simulink model "model_sim"  (Simulink 7.7)
settings: Solver=ode1  StartTime=0.0  StopTime=30  FixedStep=0.01  RelTol=1e-3
values from neighbouring files (symbols this model uses):
  sys = ss(A,B,C,D)    [model0001.m]
undefined symbols (not defined in the file or in its folder): Ainit, Binit, d1, DiscIntNeverNeededParam, sigbuilder_block, Tc
libraries: simulink x5
settings Model: Creator=User  LastModifiedBy=User
settings DataIOCC: LimitDataPoints=off  SaveFormat=StructureWithTime  SaveOutput=off  SignalLogging=off  DSMLogging=off  SaveTime=off

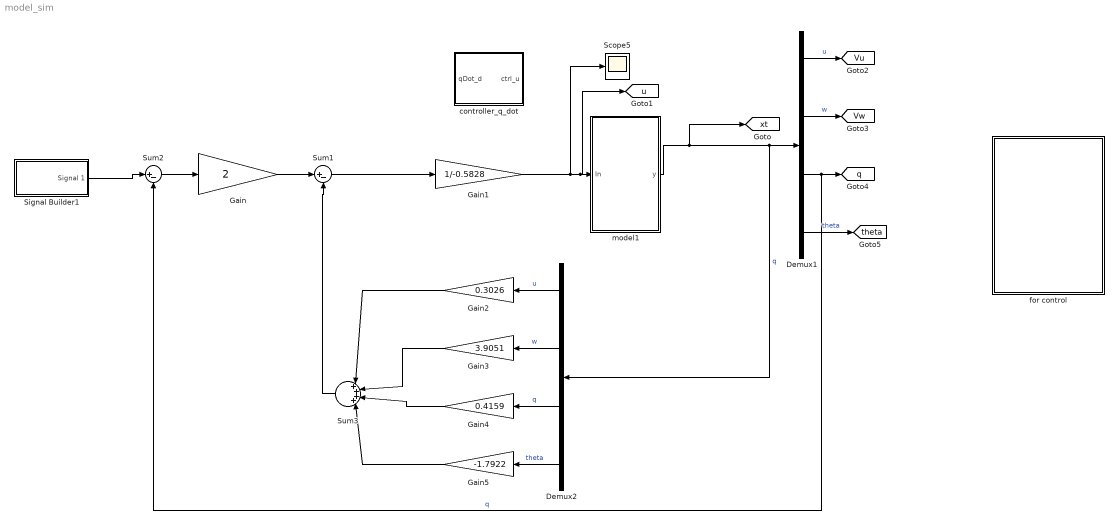
== system model_sim ==
  Demux1 : Demux
  Demux2 : Demux
  Gain : Gain  Gain=2
  Gain1 : Gain  Gain=1/-0.5828
  Gain2 : Gain  Gain=0.3026
  Gain3 : Gain  Gain=3.9051
  Gain4 : Gain  Gain=0.4159
  Gain5 : Gain  Gain=-1.7922
  Scope5 : Scope
      settings: YMin=-0.44624  YMax=0.2748
  Signal Builder1 : Subsystem  Tag=STV Subsys  LoadFcn=sigbuilder_block('load');  StartFcn=sigbuilder_block('start');  StopFcn=sigbuilder_block('stop');  ClipboardFcn=sigbuilder_block('clipboard');  mask(Sigbuilder block){}
      mask help: Create and generate interchangeable groups of signals whose waveforms are piecewise linear.
      mask init:
      | if ~strcmp(get_param(bdroot(gcbh),'SimulationStatus'),'stopped') tuvar = sigbuilder_block('maskInit'); end
      settings: CopyFcn=sigbuilder_block('copy');  DeleteFcn=sigbuilder_block('delete');  ModelCloseFcn=sigbuilder_block('modelClose');  PreSaveFcn=sigbuilder_block('preSave');  NameChangeFcn=sigbuilder_block('namechange');  OpenFcn=sigbuilder_block('open',[136.552 87.5172 549.931 396 ]);  CloseFcn=sigbuilder_block('close');
      mask Display: plot(0, 0, 100, 100,[2, 2, 32, 32, 2], [68, 8, 8, 68, 68],[32, 2], [38, 38], [32, 19, 2],[53, 60, 44], [32, 17, 17, 2],[16, 16, 31, 31]);txt = getActiveGroup(gcbh);text(2, 100, txt,'verticalAlignment', 'top');
  Sum1 : Sum  Inputs=|+-
  Sum2 : Sum  Inputs=|+-
  Sum3 : Sum  Inputs=|++++|
  controller_q_dot : Subsystem
  for control : Subsystem
  model1 : Subsystem
  tag scope: Vu=global, Vw=global, q=global, theta=global, u=global, xt=global
  wires:
  Demux1/2 -> [Vw]  "w"
  Demux2/3 -> Gain4/1  "q"
  Gain2/1 -> Sum3/1
  Demux2/1 -> Gain2/1  "u"
  Gain4/1 -> Sum3/3
  Gain5/1 -> Sum3/4
  Gain3/1 -> Sum3/2
  Demux2/4 -> Gain5/1  "theta"
  Demux1/1 -> [Vu]  "u"
  Sum2/1 -> Gain/1
  model1/1(y) -> [xt], Demux1/1, Demux2/1  "q"
  Demux2/2 -> Gain3/1  "w"
  Demux1/3 -> Sum2/2, [q]  "q"
  Demux1/4 -> [theta]  "theta"
  Gain/1 -> Sum1/1
  Sum3/1 -> Sum1/2
  Sum1/1 -> Gain1/1
  Signal Builder1/1(Signal 1) -> Sum2/1
  Gain1/1 -> [u], model1/1(In), Scope5/1

== system model_sim/Signal Builder1 ==
  Demux : Demux  Tag=STV Demux  Outputs=1
  FromWs : FromWorkspace  Tag=STV FromWs  VariableName=tuvar  SampleTime=0  SigBuilderData=DataTag0  VnvData=DataTag1
      SigBuilderData=|
      | common.afterFinalStr = 'Extrapolate'
      | common.sampleTime = 0
      | dataSet.timeRange = [0 30]
      | dataSet.name = 'Group 1'
      | sbobj.Groups.Name = 'Group 1'
      | sbobj.Groups.Signals.Name = 'Signal 1'
      | sbobj.Groups.Signals.XData = [0 0.6 0.6 1.25 1.25 1.8 1.8 2.65 2.65 3.25 3.25 3.75 3.75 4.3 4.3 5.1 5.1 6 6 6.55 6.55 7.85 7.85 8.3 8.3 8.95 8.95 9.45 9.45 10.3 10.3 10.95 10.95 11.6 11.6 12.05 12.05 13.15 13.15 14.1 14.1 15.15 15.15 15.85 15.85 16.25 16.75 17.6 18.1 18.1 19.15 19.15 19.8 19.8 20.45 20.45 21.3 21.3 21.95 21.95 23.05 23.05 23.85 23.85 24.5 24.5 25.15 25.15 25.6 25.6 26.2 26.2 26.65 26.65 27.2 27.2 27.95 27.95 28.6 28.6 29.25 29.25 30]
      | sbobj.Groups.Signals.YData = [-0.4 -0.4 -0.105 -0.105 0.53 0.53 0.17 0.17 -0.075 -0.075 0.26 0.26 -0.33 -0.33 0.055 0.055 0.405 0.405 0.29 0.29 0.255 0.255 -0.05 -0.05 0.39 0.39 -0.25 -0.25 0.135 0.135 -0.345 -0.345 -0.055 -0.055 0.19 0.19 0.31 0.31 0.445 0.445 0 0 -0.28 -0.28 0.12 0.115 0.245 -0.02 0 -0.53 -0.53 0.46 0.46 -0.11 -0.11 0.01 0.01 0.1 0.1 0.5 0.5 -0.19 -0.19 0.24 0.24 -0.09 -0.09 0 0 -0.355 -0.355 -0.115 -0.115 0.065 0.065 0.025 0.025 -0.16 -0.16 0.075 0.075 -0.04 -0.04]
      | sbobj.Groups.TimeRange = [0 30]
  Signal 1 : Outport  Tag=STV Outport
  wires:
  FromWs/1 -> Demux/1
  Demux/1 -> Signal 1/1

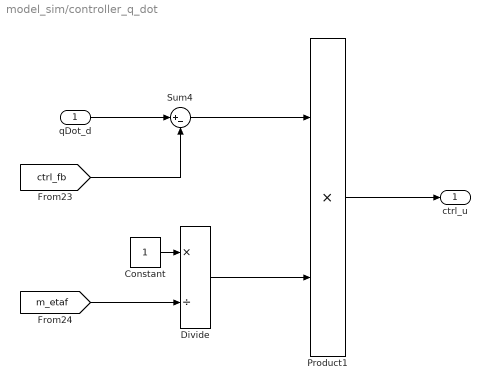
== system model_sim/controller_q_dot ==
  qDot_d : Inport
  Constant : Constant
  Divide : Product  Inputs=*/
  Product1 : Product
  Sum4 : Sum  Inputs=|+-
  ctrl_u : Outport
  wires:
  Sum4/1 -> Product1/1
  Product1/1 -> ctrl_u/1
  [m_etaf] -> Divide/2
  Divide/1 -> Product1/2
  [ctrl_fb] -> Sum4/2
  qDot_d/1 -> Sum4/1
  Constant/1 -> Divide/1

== system model_sim/for control ==
  DI_Control : Subsystem
  incremental : Subsystem
  tag scope: ctrl_fb=global
  wires:
  [xt] -> incremental/1(xt)
  [u] -> incremental/3(u)
  DI_Control/1(control_fb) -> [ctrl_fb]
  [xt1] -> incremental/2(xt1)

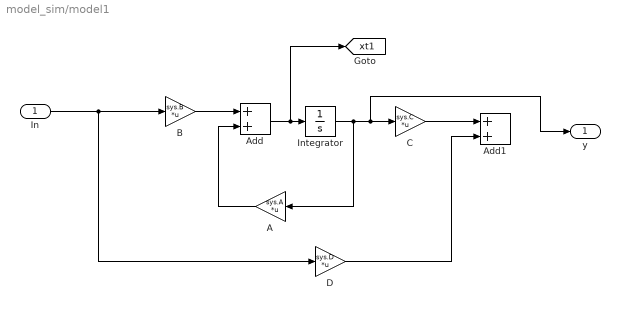
== system model_sim/model1 ==
  In : Inport
  A : Gain  Gain=sys.A  Multiplication=Matrix(K*u)
  Add : Sum
  Add1 : Sum
  B : Gain  Gain=sys.B  Multiplication=Matrix(K*u)
  C : Gain  Gain=sys.C  Multiplication=Matrix(K*u)
  D : Gain  Gain=sys.D  Multiplication=Matrix(K*u)
  Integrator : Integrator
  y : Outport
  tag scope: xt1=global
  wires:
  B/1 -> Add/1
  Integrator/1 -> A/1, y/1, C/1
  Add/1 -> Integrator/1, [xt1]
  C/1 -> Add1/1
  In/1 -> B/1, D/1
  D/1 -> Add1/2
  A/1 -> Add/2

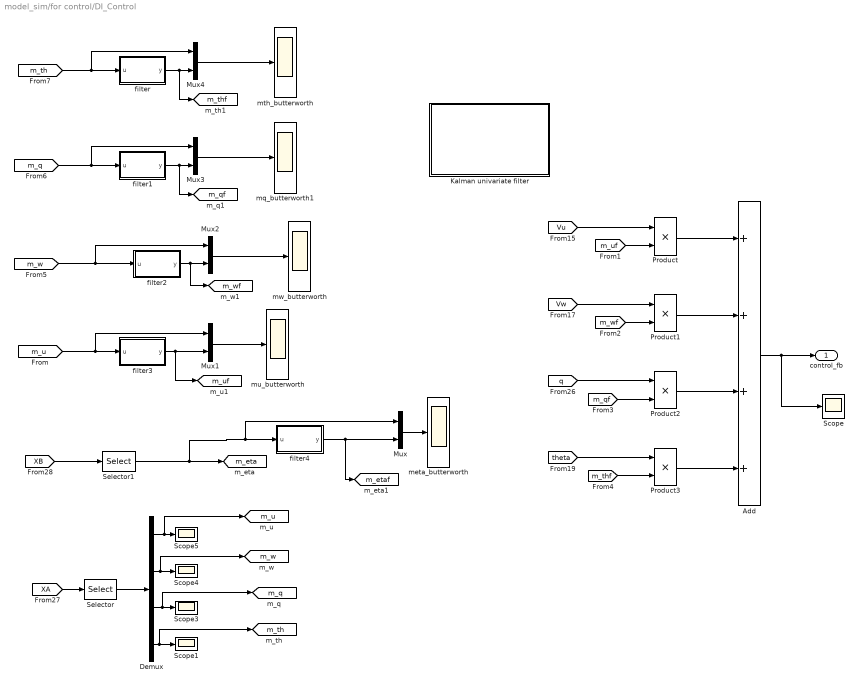
== system model_sim/for control/DI_Control ==
  Add : Sum  Inputs=++++
  Demux : Demux
  Kalman univariate filter : Subsystem
  Mux{,1..4} (5 alike) : Mux  Inputs=2
  Product{,1..3} (4 alike) : Product
  Scope{,1,3..5} (5 alike) : Scope
      Scope settings: YMin=-0.09848  YMax=0.08425  SaveName=ScopeData11
      Scope1 settings: YMin=-2.43463  YMax=-1.68294  SaveName=ScopeData23
      Scope3 settings: YMin=0.37059  YMax=0.82372  SaveName=ScopeData24
      Scope4 settings: YMin=3.69303  YMax=5.18093  SaveName=ScopeData25
      Scope5 settings: YMin=0.11118  YMax=0.81384  SaveName=ScopeData26
  Selector : Selector  NumberOfDimensions=2  InputPortWidth=3  IndexOptions=Index vector (dialog),Index vector (dialog)  Indices=3,[1 2 3 4]  OutputSizes=1,1
  Selector1 : Selector  InputPortWidth=4  IndexOptions=Index vector (dialog)  Indices=3  OutputSizes=1
  filter : Subsystem
  filter1 : Subsystem
  filter2 : Subsystem
  filter3 : Subsystem
  filter4 : Subsystem
  meta_butterworth : Scope
      settings: YMin=-0.60773  YMax=-0.35841  SaveName=ScopeData6
  mq_butterworth1 : Scope
      settings: YMin=3.69303  YMax=5.18093  SaveName=ScopeData10
  mth_butterworth : Scope
      settings: YMin=3.69303  YMax=5.18093  SaveName=ScopeData14
  mu_butterworth : Scope
      settings: YMin=0.19635  YMax=0.80437  SaveName=ScopeData2
  mw_butterworth : Scope
      settings: YMin=3.69303  YMax=5.18093  SaveName=ScopeData4
  control_fb : Outport
  tag scope: m_eta=global, m_etaf=global, m_q=global, m_qf=global, m_th=global, m_thf=global, m_u=global, m_uf=global, m_w=global, m_wf=global
  wires:
  [XA] -> Selector/1
  [theta] -> Product3/1
  [Vu] -> Product/1
  [q] -> Product2/1
  [XB] -> Selector1/1
  [Vw] -> Product1/1
  Selector/1 -> Demux/1
  Selector1/1 -> Mux/1, filter4/1(u), [m_eta]
  Demux/2 -> Scope4/1, [m_w]
  Demux/3 -> Scope3/1, [m_q]
  Demux/4 -> [m_th], Scope1/1
  [m_uf] -> Product/2
  [m_wf] -> Product1/2
  [m_qf] -> Product2/2
  [m_thf] -> Product3/2
  Product/1 -> Add/1
  Product1/1 -> Add/2
  Product2/1 -> Add/3
  Product3/1 -> Add/4
  Add/1 -> Scope/1, control_fb/1
  filter4/1(y) -> [m_etaf], Mux/2
  Demux/1 -> Scope5/1, [m_u]
  Mux/1 -> meta_butterworth/1
  [m_u] -> Mux1/1, filter3/1(u)
  Mux1/1 -> mu_butterworth/1
  filter3/1(y) -> Mux1/2, [m_uf]
  [m_w] -> Mux2/1, filter2/1(u)
  Mux2/1 -> mw_butterworth/1
  filter2/1(y) -> Mux2/2, [m_wf]
  [m_q] -> Mux3/1, filter1/1(u)
  Mux3/1 -> mq_butterworth1/1
  filter1/1(y) -> Mux3/2, [m_qf]
  [m_th] -> Mux4/1, filter/1(u)
  Mux4/1 -> mth_butterworth/1
  filter/1(y) -> Mux4/2, [m_thf]

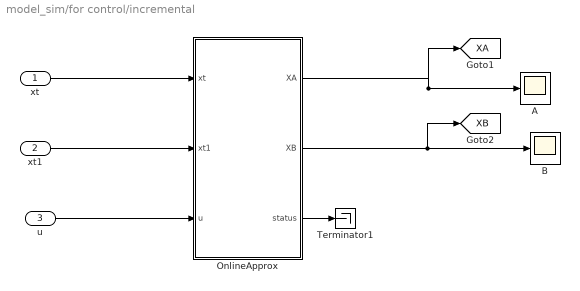
== system model_sim/for control/incremental ==
  xt : Inport
  xt1 : Inport  Port=2
  u : Inport  Port=3
  "A  " : Scope
      settings: YMin=-1.60203  YMax=1.90229  SaveName=ScopeData4
  "B  " : Scope
      settings: YMin=-0.6917  YMax=0.17944
  OnlineApprox : Subsystem
  Terminator1 : Terminator
  tag scope: XA=global, XB=global
  wires:
  OnlineApprox/1(XA) -> [XA], "A  "/1
  OnlineApprox/2(XB) -> [XB], "B  "/1
  xt1/1 -> OnlineApprox/2(xt1)
  xt/1 -> OnlineApprox/1(xt)
  u/1 -> OnlineApprox/3(u)
  OnlineApprox/3(status) -> Terminator1/1

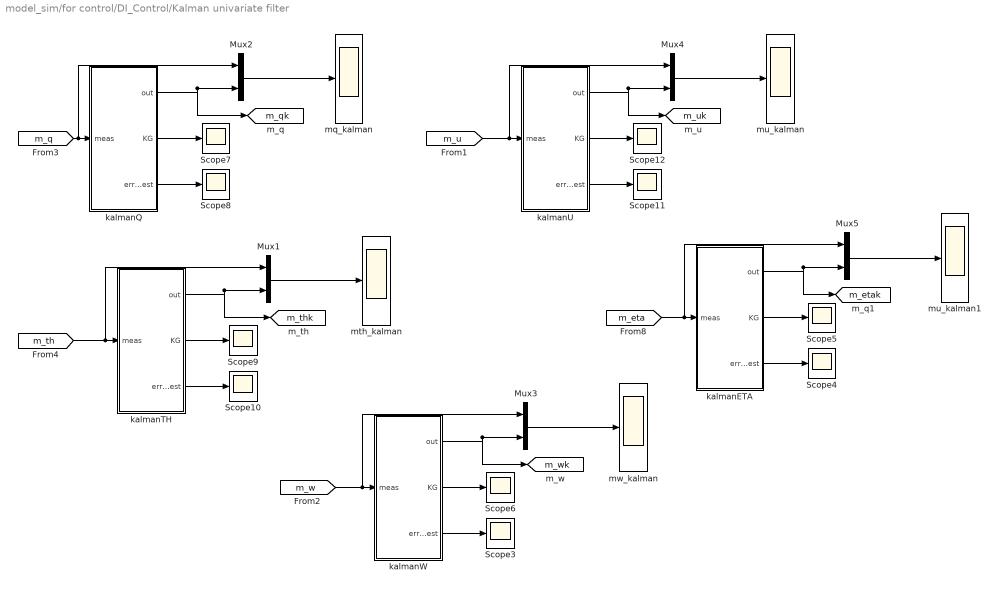
== system model_sim/for control/DI_Control/Kalman univariate filter ==
  Mux{1..5} (5 alike) : Mux  Inputs=2
  Scope{3..12} (10 alike) : Scope
      Scope10 settings: YMin=-0.05948  YMax=0.53571  SaveName=ScopeData16
      Scope11 settings: YMin=-0.05948  YMax=0.53571  SaveName=ScopeData21
      Scope12 settings: YMin=-0.00332  YMax=0.00334  SaveName=ScopeData22
      Scope3 settings: YMin=-0.05948  YMax=0.53571  SaveName=ScopeData3
      Scope4 settings: YMin=-0.05948  YMax=0.53571  SaveName=ScopeData7
      Scope5 settings: YMin=-0.00332  YMax=0.00334  SaveName=ScopeData12
      Scope6 settings: YMin=-0.00332  YMax=0.00334  SaveName=ScopeData19
      Scope7 settings: YMin=-0.00332  YMax=0.00334  SaveName=ScopeData4
      Scope8 settings: YMin=-0.05948  YMax=0.53571  SaveName=ScopeData5
      Scope9 settings: YMin=-0.00332  YMax=0.00334  SaveName=ScopeData17
  kalmanETA : Stateflow chart  TreatAsAtomicUnit=on
  kalmanQ : Stateflow chart  TreatAsAtomicUnit=on
  kalmanTH : Stateflow chart  TreatAsAtomicUnit=on
  kalmanU : Stateflow chart  TreatAsAtomicUnit=on
  kalmanW : Stateflow chart  TreatAsAtomicUnit=on
  mq_kalman : Scope
      settings: YMin=3.69303  YMax=5.18093  SaveName=ScopeData15
  mth_kalman : Scope
      settings: YMin=3.69303  YMax=5.18093  SaveName=ScopeData18
  mu_kalman : Scope
      settings: YMin=3.69303  YMax=5.18093  SaveName=ScopeData27
  mu_kalman1 : Scope
      settings: YMin=3.69303  YMax=5.18093  SaveName=ScopeData28
  mw_kalman : Scope
      settings: YMin=3.69303  YMax=5.18093  SaveName=ScopeData20
  tag scope: m_etak=global, m_qk=global, m_thk=global, m_uk=global, m_wk=global
  wires:
  kalmanQ/3(error_est) -> Scope8/1
  kalmanQ/2(KG) -> Scope7/1
  kalmanQ/1(out) -> [m_qk], Mux2/2
  [m_q] -> kalmanQ/1(meas), Mux2/1
  Mux2/1 -> mq_kalman/1
  kalmanTH/3(error_est) -> Scope10/1
  kalmanTH/2(KG) -> Scope9/1
  kalmanTH/1(out) -> Mux1/2, [m_thk]
  [m_th] -> Mux1/1, kalmanTH/1(meas)
  Mux1/1 -> mth_kalman/1
  kalmanW/3(error_est) -> Scope3/1
  kalmanW/2(KG) -> Scope6/1
  kalmanW/1(out) -> Mux3/2, [m_wk]
  [m_w] -> kalmanW/1(meas), Mux3/1
  Mux3/1 -> mw_kalman/1
  kalmanU/3(error_est) -> Scope11/1
  kalmanU/2(KG) -> Scope12/1
  kalmanU/1(out) -> Mux4/2, [m_uk]
  [m_u] -> Mux4/1, kalmanU/1(meas)
  Mux4/1 -> mu_kalman/1
  kalmanETA/3(error_est) -> Scope4/1
  kalmanETA/2(KG) -> Scope5/1
  kalmanETA/1(out) -> Mux5/2, [m_etak]
  [m_eta] -> kalmanETA/1(meas), Mux5/1
  Mux5/1 -> mu_kalman1/1

== system model_sim/for control/DI_Control/filter ==
  u : Inport
  1/T : Product  Inputs=/*
  Enable/Disable  time constant : Subsystem
  Sum : Sum  Inputs=-+|
  integral : Subsystem
  y : Outport
  wires:
  integral/1(y) -> y/1, Enable/Disable  time constant/1(x), Sum/1
  Enable/Disable  time constant/2(reset) -> integral/2(Reset)
  1/T/1 -> integral/1(u)
  Enable/Disable  time constant/1(max(T,Ts)) -> 1/T/1
  Sum/1 -> 1/T/2
  u/1 -> Sum/2, integral/3(x0)

== system model_sim/for control/DI_Control/filter1 ==
  u : Inport
  1/T : Product  Inputs=/*
  Enable/Disable  time constant : Subsystem
  Sum : Sum  Inputs=-+|
  integral : Subsystem
  y : Outport
  wires:
  u/1 -> integral/3(x0), Sum/2
  Sum/1 -> 1/T/2
  Enable/Disable  time constant/1(max(T,Ts)) -> 1/T/1
  1/T/1 -> integral/1(u)
  Enable/Disable  time constant/2(reset) -> integral/2(Reset)
  integral/1(y) -> Sum/1, Enable/Disable  time constant/1(x), y/1

== system model_sim/for control/DI_Control/filter2 ==
  u : Inport
  1/T : Product  Inputs=/*
  Enable/Disable  time constant : Subsystem
  Sum : Sum  Inputs=-+|
  integral : Subsystem
  y : Outport
  wires:
  integral/1(y) -> y/1, Enable/Disable  time constant/1(x), Sum/1
  Enable/Disable  time constant/2(reset) -> integral/2(Reset)
  1/T/1 -> integral/1(u)
  Enable/Disable  time constant/1(max(T,Ts)) -> 1/T/1
  Sum/1 -> 1/T/2
  u/1 -> Sum/2, integral/3(x0)

== system model_sim/for control/DI_Control/filter3 ==
  u : Inport
  1/T : Product  Inputs=/*
  Enable/Disable  time constant : Subsystem
  Sum : Sum  Inputs=-+|
  integral : Subsystem
  y : Outport
  wires:
  u/1 -> integral/3(x0), Sum/2
  Sum/1 -> 1/T/2
  Enable/Disable  time constant/1(max(T,Ts)) -> 1/T/1
  1/T/1 -> integral/1(u)
  Enable/Disable  time constant/2(reset) -> integral/2(Reset)
  integral/1(y) -> Sum/1, Enable/Disable  time constant/1(x), y/1

== system model_sim/for control/DI_Control/filter4 ==
  u : Inport
  1/T : Product  Inputs=/*
  Enable/Disable  time constant : Subsystem
  Sum : Sum  Inputs=-+|
  integral : Subsystem
  y : Outport
  wires:
  integral/1(y) -> y/1, Enable/Disable  time constant/1(x), Sum/1
  Enable/Disable  time constant/2(reset) -> integral/2(Reset)
  1/T/1 -> integral/1(u)
  Enable/Disable  time constant/1(max(T,Ts)) -> 1/T/1
  Sum/1 -> 1/T/2
  u/1 -> Sum/2, integral/3(x0)

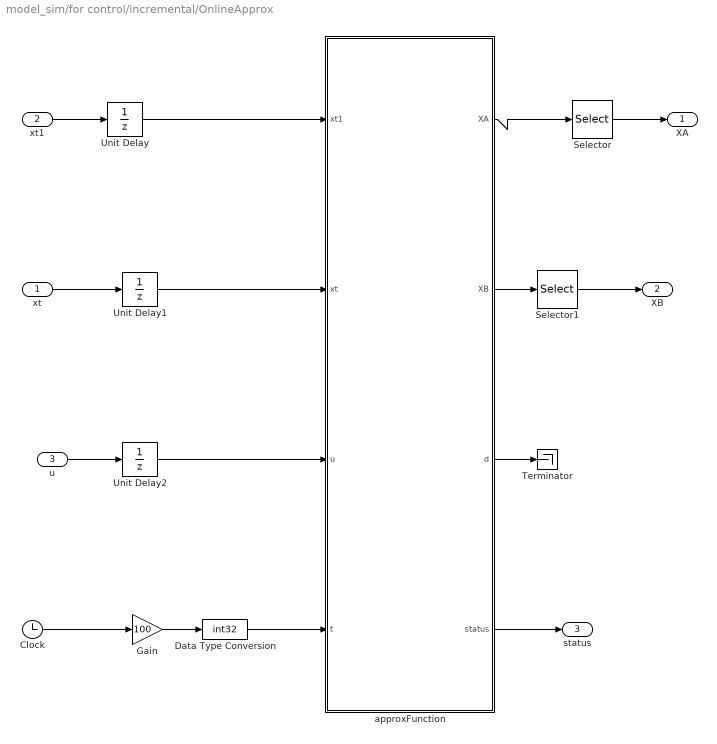
== system model_sim/for control/incremental/OnlineApprox ==
  xt : Inport
  xt1 : Inport  Port=2
  u : Inport  Port=3
  Clock : Clock
      settings: Decimation=10
  Data Type Conversion : DataTypeConversion  OutDataTypeStr=int32
  Gain : Gain  Gain=100
  Selector : Selector  NumberOfDimensions=2  InputPortWidth=3  IndexOptions=Index vector (dialog),Index vector (dialog)  Indices=[1 2 3 4],[1 2 3 4]  OutputSizes=1,1
  Selector1 : Selector  NumberOfDimensions=2  InputPortWidth=3  IndexOptions=Index vector (dialog),Index vector (dialog)  Indices=[1 2 3 4],[1]  OutputSizes=1,1
  Terminator : Terminator
  Unit Delay : UnitDelay  SampleTime=-1
  Unit Delay1 : UnitDelay  SampleTime=-1
  Unit Delay2 : UnitDelay  SampleTime=-1
  approxFunction : Stateflow chart  TreatAsAtomicUnit=on
  XA : Outport
  XB : Outport  Port=2
  status : Outport  Port=3
  wires:
  Data Type Conversion/1 -> approxFunction/4(t)
  Clock/1 -> Gain/1
  Gain/1 -> Data Type Conversion/1
  approxFunction/2(XB) -> Selector1/1
  xt1/1 -> Unit Delay/1
  xt/1 -> Unit Delay1/1
  u/1 -> Unit Delay2/1
  approxFunction/1(XA) -> Selector/1
  Selector/1 -> XA/1
  Selector1/1 -> XB/1
  Unit Delay2/1 -> approxFunction/3(u)
  Unit Delay1/1 -> approxFunction/2(xt)
  Unit Delay/1 -> approxFunction/1(xt1)
  approxFunction/3(d) -> Terminator/1
  approxFunction/4(status) -> status/1

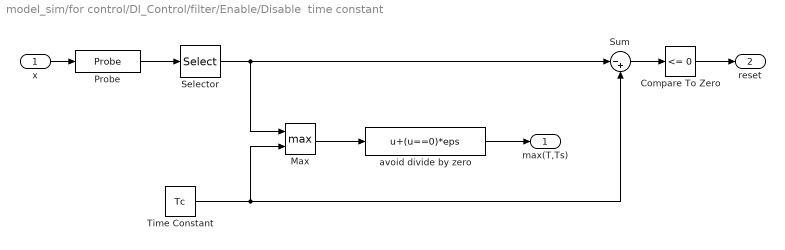
== system model_sim/for control/DI_Control/filter/Enable/Disable  time constant ==
  x : Inport
  Compare To Zero : simulink/Logic and Bit Operations/Compare To Zero  SystemSampleTime=-1  relop=<=  LogicOutDataTypeMode=uint8
  Max : MinMax  Function=max  Inputs=2
  Probe : Probe  ProbeWidth=off  ProbeComplexSignal=off
  Selector : Selector  InputPortWidth=2  IndexOptions=Index vector (dialog)  Indices=1  OutputSizes=1
  Sum : Sum  Inputs=|-+
  Time Constant : Constant  Value=Tc
  avoid divide by zero : Fcn  Expr=u+(u==0)*eps
  max(T,Ts) : Outport
  reset : Outport  Port=2
  wires:
  Max/1 -> avoid divide by zero/1
  Selector/1 -> Max/1, Sum/1
  avoid divide by zero/1 -> max(T,Ts)/1
  Time Constant/1 -> Max/2, Sum/2
  Compare To Zero/1 -> reset/1
  Sum/1 -> Compare To Zero/1
  x/1 -> Probe/1
  Probe/1 -> Selector/1

== system model_sim/for control/DI_Control/filter/integral ==
  u : Inport
  Reset : Inport  Port=2
  x0 : Inport  Port=3
  Discrete-Time Integrator : DiscreteIntegrator  ExternalReset=level  InitialConditionSource=external  SampleTime=-1  ICPrevOutput=DiscIntNeverNeededParam  ICPrevScaledInput=DiscIntNeverNeededParam
  Saturation : Saturate  UpperLimit=inf  LowerLimit=-inf
  y : Outport
  wires:
  u/1 -> Discrete-Time Integrator/1
  Reset/1 -> Discrete-Time Integrator/2
  Discrete-Time Integrator/1 -> Saturation/1
  x0/1 -> Discrete-Time Integrator/3
  Saturation/1 -> y/1

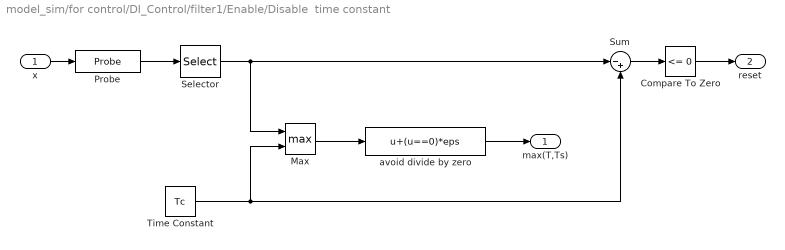
== system model_sim/for control/DI_Control/filter1/Enable/Disable  time constant ==
  x : Inport
  Compare To Zero : simulink/Logic and Bit Operations/Compare To Zero  SystemSampleTime=-1  relop=<=  LogicOutDataTypeMode=uint8
  Max : MinMax  Function=max  Inputs=2
  Probe : Probe  ProbeWidth=off  ProbeComplexSignal=off
  Selector : Selector  InputPortWidth=2  IndexOptions=Index vector (dialog)  Indices=1  OutputSizes=1
  Sum : Sum  Inputs=|-+
  Time Constant : Constant  Value=Tc
  avoid divide by zero : Fcn  Expr=u+(u==0)*eps
  max(T,Ts) : Outport
  reset : Outport  Port=2
  wires:
  Probe/1 -> Selector/1
  x/1 -> Probe/1
  Sum/1 -> Compare To Zero/1
  Compare To Zero/1 -> reset/1
  Time Constant/1 -> Sum/2, Max/2
  avoid divide by zero/1 -> max(T,Ts)/1
  Selector/1 -> Sum/1, Max/1
  Max/1 -> avoid divide by zero/1

== system model_sim/for control/DI_Control/filter1/integral ==
  u : Inport
  Reset : Inport  Port=2
  x0 : Inport  Port=3
  Discrete-Time Integrator : DiscreteIntegrator  ExternalReset=level  InitialConditionSource=external  SampleTime=-1  ICPrevOutput=DiscIntNeverNeededParam  ICPrevScaledInput=DiscIntNeverNeededParam
  Saturation : Saturate  UpperLimit=inf  LowerLimit=-inf
  y : Outport
  wires:
  Saturation/1 -> y/1
  x0/1 -> Discrete-Time Integrator/3
  Discrete-Time Integrator/1 -> Saturation/1
  Reset/1 -> Discrete-Time Integrator/2
  u/1 -> Discrete-Time Integrator/1

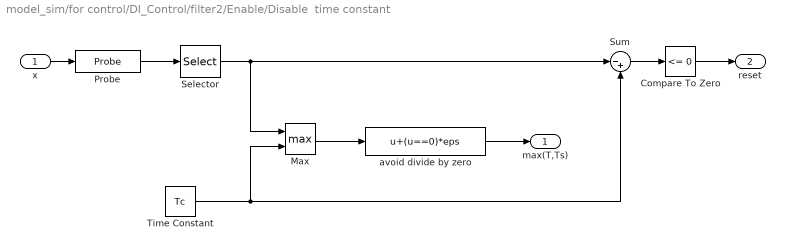
== system model_sim/for control/DI_Control/filter2/Enable/Disable  time constant ==
  x : Inport
  Compare To Zero : simulink/Logic and Bit Operations/Compare To Zero  SystemSampleTime=-1  relop=<=  LogicOutDataTypeMode=uint8
  Max : MinMax  Function=max  Inputs=2
  Probe : Probe  ProbeWidth=off  ProbeComplexSignal=off
  Selector : Selector  InputPortWidth=2  IndexOptions=Index vector (dialog)  Indices=1  OutputSizes=1
  Sum : Sum  Inputs=|-+
  Time Constant : Constant  Value=Tc
  avoid divide by zero : Fcn  Expr=u+(u==0)*eps
  max(T,Ts) : Outport
  reset : Outport  Port=2
  wires:
  Max/1 -> avoid divide by zero/1
  Selector/1 -> Max/1, Sum/1
  avoid divide by zero/1 -> max(T,Ts)/1
  Time Constant/1 -> Max/2, Sum/2
  Compare To Zero/1 -> reset/1
  Sum/1 -> Compare To Zero/1
  x/1 -> Probe/1
  Probe/1 -> Selector/1

== system model_sim/for control/DI_Control/filter2/integral ==
  u : Inport
  Reset : Inport  Port=2
  x0 : Inport  Port=3
  Discrete-Time Integrator : DiscreteIntegrator  ExternalReset=level  InitialConditionSource=external  SampleTime=-1  ICPrevOutput=DiscIntNeverNeededParam  ICPrevScaledInput=DiscIntNeverNeededParam
  Saturation : Saturate  UpperLimit=inf  LowerLimit=-inf
  y : Outport
  wires:
  u/1 -> Discrete-Time Integrator/1
  Reset/1 -> Discrete-Time Integrator/2
  Discrete-Time Integrator/1 -> Saturation/1
  x0/1 -> Discrete-Time Integrator/3
  Saturation/1 -> y/1

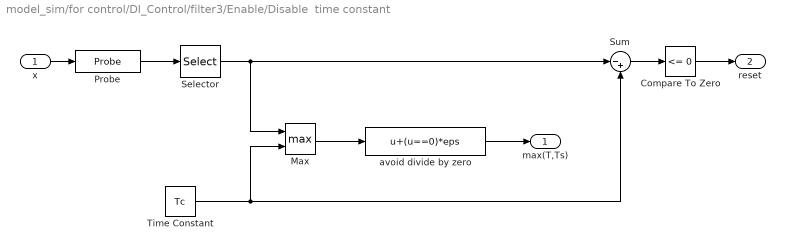
== system model_sim/for control/DI_Control/filter3/Enable/Disable  time constant ==
  x : Inport
  Compare To Zero : simulink/Logic and Bit Operations/Compare To Zero  SystemSampleTime=-1  relop=<=  LogicOutDataTypeMode=uint8
  Max : MinMax  Function=max  Inputs=2
  Probe : Probe  ProbeWidth=off  ProbeComplexSignal=off
  Selector : Selector  InputPortWidth=2  IndexOptions=Index vector (dialog)  Indices=1  OutputSizes=1
  Sum : Sum  Inputs=|-+
  Time Constant : Constant  Value=Tc
  avoid divide by zero : Fcn  Expr=u+(u==0)*eps
  max(T,Ts) : Outport
  reset : Outport  Port=2
  wires:
  Probe/1 -> Selector/1
  x/1 -> Probe/1
  Sum/1 -> Compare To Zero/1
  Compare To Zero/1 -> reset/1
  Time Constant/1 -> Sum/2, Max/2
  avoid divide by zero/1 -> max(T,Ts)/1
  Selector/1 -> Sum/1, Max/1
  Max/1 -> avoid divide by zero/1

== system model_sim/for control/DI_Control/filter3/integral ==
  u : Inport
  Reset : Inport  Port=2
  x0 : Inport  Port=3
  Discrete-Time Integrator : DiscreteIntegrator  ExternalReset=level  InitialConditionSource=external  SampleTime=-1  ICPrevOutput=DiscIntNeverNeededParam  ICPrevScaledInput=DiscIntNeverNeededParam
  Saturation : Saturate  UpperLimit=inf  LowerLimit=-inf
  y : Outport
  wires:
  Saturation/1 -> y/1
  x0/1 -> Discrete-Time Integrator/3
  Discrete-Time Integrator/1 -> Saturation/1
  Reset/1 -> Discrete-Time Integrator/2
  u/1 -> Discrete-Time Integrator/1

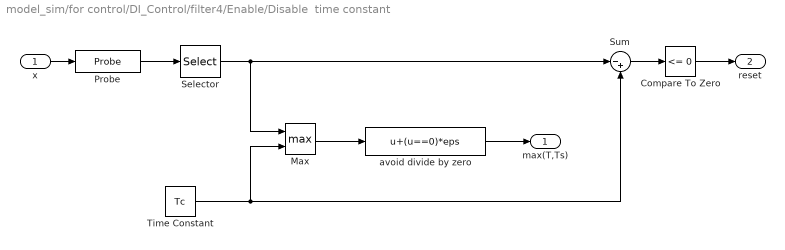
== system model_sim/for control/DI_Control/filter4/Enable/Disable  time constant ==
  x : Inport
  Compare To Zero : simulink/Logic and Bit Operations/Compare To Zero  SystemSampleTime=-1  relop=<=  LogicOutDataTypeMode=uint8
  Max : MinMax  Function=max  Inputs=2
  Probe : Probe  ProbeWidth=off  ProbeComplexSignal=off
  Selector : Selector  InputPortWidth=2  IndexOptions=Index vector (dialog)  Indices=1  OutputSizes=1
  Sum : Sum  Inputs=|-+
  Time Constant : Constant  Value=Tc
  avoid divide by zero : Fcn  Expr=u+(u==0)*eps
  max(T,Ts) : Outport
  reset : Outport  Port=2
  wires:
  Max/1 -> avoid divide by zero/1
  Selector/1 -> Max/1, Sum/1
  avoid divide by zero/1 -> max(T,Ts)/1
  Time Constant/1 -> Max/2, Sum/2
  Compare To Zero/1 -> reset/1
  Sum/1 -> Compare To Zero/1
  x/1 -> Probe/1
  Probe/1 -> Selector/1

== system model_sim/for control/DI_Control/filter4/integral ==
  u : Inport
  Reset : Inport  Port=2
  x0 : Inport  Port=3
  Discrete-Time Integrator : DiscreteIntegrator  ExternalReset=level  InitialConditionSource=external  SampleTime=-1  ICPrevOutput=DiscIntNeverNeededParam  ICPrevScaledInput=DiscIntNeverNeededParam
  Saturation : Saturate  UpperLimit=inf  LowerLimit=-inf
  y : Outport
  wires:
  u/1 -> Discrete-Time Integrator/1
  Reset/1 -> Discrete-Time Integrator/2
  Discrete-Time Integrator/1 -> Saturation/1
  x0/1 -> Discrete-Time Integrator/3
  Saturation/1 -> y/1

== matlab function for control/DI_Control/Kalman univariate filter/kalmanQ ==
  settings: updateMethod=DISCRETE  sampleTime=0.01
  data: meas input double; out output double; KG output double; error_est output double
function [out, KG, error_est] = KALMAN(meas)
%#codegen

persistent EST E_est E_meas EST_prev E_est_prev
if isempty(EST)
   E_est = 10;
   E_est_prev = 10;
   E_meas = 0.5;
end

KG = (E_est/(E_est + E_meas));

if isempty(EST_prev)
    EST_prev = meas;
    EST = EST_prev + KG*(meas - EST_prev);
else
    EST = (EST_prev + KG*(meas - EST_prev));
end

EST_prev = EST;

E_est = (1-KG)*(E_est_prev);

E_est_prev = E_est;

error_est = E_est;

out = EST;
end

== matlab function for control/DI_Control/Kalman univariate filter/kalmanTH ==
  settings: updateMethod=DISCRETE  sampleTime=0.01
  data: meas input double; out output double; KG output double; error_est output double
function [out, KG, error_est] = KALMAN(meas)
%#codegen

persistent EST E_est E_meas EST_prev E_est_prev
if isempty(EST)
   E_est = 10;
   E_est_prev = 10;
   E_meas = 0.5;
end

KG = (E_est/(E_est + E_meas));

if isempty(EST_prev)
    EST_prev = meas;
    EST = EST_prev + KG*(meas - EST_prev);
else
    EST = (EST_prev + KG*(meas - EST_prev));
end

EST_prev = EST;

E_est = (1-KG)*(E_est_prev);

E_est_prev = E_est;

error_est = E_est;

out = EST;
end

== matlab function for control/DI_Control/Kalman univariate filter/kalmanW ==
  settings: updateMethod=DISCRETE  sampleTime=0.01
  data: meas input double; out output double; KG output double; error_est output double
function [out, KG, error_est] = KALMAN(meas)
%#codegen

persistent EST E_est E_meas EST_prev E_est_prev
if isempty(EST)
   E_est = 10;
   E_est_prev = 10;
   E_meas = 0.5;
end

KG = (E_est/(E_est + E_meas));

if isempty(EST_prev)
    EST_prev = meas;
    EST = EST_prev + KG*(meas - EST_prev);
else
    EST = (EST_prev + KG*(meas - EST_prev));
end

EST_prev = EST;

E_est = (1-KG)*(E_est_prev);

E_est_prev = E_est;

error_est = E_est;

out = EST;
end

== matlab function for control/DI_Control/Kalman univariate filter/kalmanU ==
  settings: updateMethod=DISCRETE  sampleTime=0.01
  data: meas input double; out output double; KG output double; error_est output double
function [out, KG, error_est] = KALMAN(meas)
%#codegen

persistent EST E_est E_meas EST_prev E_est_prev
if isempty(EST)
   E_est = 10;
   E_est_prev = 10;
   E_meas = 0.5;
end

KG = (E_est/(E_est + E_meas));

if isempty(EST_prev)
    EST_prev = meas;
    EST = EST_prev + KG*(meas - EST_prev);
else
    EST = (EST_prev + KG*(meas - EST_prev));
end

EST_prev = EST;

E_est = (1-KG)*(E_est_prev);

E_est_prev = E_est;

error_est = E_est;

out = EST;
end

== matlab function for control/DI_Control/Kalman univariate filter/kalmanETA ==
  settings: updateMethod=DISCRETE  sampleTime=0.01
  data: meas input double; out output double; KG output double; error_est output double
function [out, KG, error_est] = KALMAN(meas)
%#codegen

persistent EST E_est E_meas EST_prev E_est_prev
if isempty(EST)
   E_est = 10;
   E_est_prev = 10;
   E_meas = 0.5;
end

KG = (E_est/(E_est + E_meas));

if isempty(EST_prev)
    EST_prev = meas;
    EST = EST_prev + KG*(meas - EST_prev);
else
    EST = (EST_prev + KG*(meas - EST_prev));
end

EST_prev = EST;

E_est = (1-KG)*(E_est_prev);

E_est_prev = E_est;

error_est = E_est;

out = EST;
end

== matlab function for control/incremental/OnlineApprox/approxFunction ==
  settings: updateMethod=DISCRETE  sampleTime=0.01
  data Ainit settings: description=Offline approximation of matrix A (8 x 8)
  data Binit settings: description=Initial offline estimation of matrix B (8 x 4)
  data: xt1 input double; xt input double; u input double; XA output double size=[4 4]; XB output double size=[4 1]; t input double; d output double; status output double; Ainit parameter double size=[4 4]; Binit parameter double size=[4 1]; d1 parameter double
function [XA, XB, d, status] = compute(xt1, xt, u, t, Ainit, Binit, d1)
%#codegen

r = 301;
n = 4;
m = 1;
% d1 = 0.01;


t = t+1;
nn = n + m;

d = d1;
persistent Ap;
persistent bp;
persistent XA_prev;
persistent XB_prev;
persistent old_data;

if isempty(Ap)
    Ap =  zeros(r,nn);
    bp = zeros(r, n);
end

XA_init = Ainit;
XB_init = Binit;



if t <= r
    Ap(t,:) = [xt;u];
    bp(t,:) = xt1;
    
    XA =  XA_init;

    XB = XB_init;
    status = 404;
    old_data = Ap(3,:);
    
else
    
    Ap = circshift(Ap, r-1);
    Ap(end,:) = [xt;u];
    
    bp = circshift(bp, r-1);
    bp(end,:) = xt1;
    
    if isempty(old_data)
        old_data = Ap(3,:);
    end
    
%         if rank(Ap(fix(r/2):end, :)) == size(Ap,2)

    if rank(Ap(fix(r/r):end, :)) == size(Ap,2)
        if mod(double(t)/100, d) == 0
            E = Ap - repmat(old_data,size(Ap,1),1);
            old_data = Ap(end,:);
            EE = Ap;
            status = 400;
            XX = (EE' * EE)^(-1) * EE' *bp;
            X2 = XX';
            XA = X2(:,1:n);
            XB = X2(:,n+1:end);
            XA_prev = XA;
            XB_prev = XB;
        else
            
            if isempty(XA_prev)
                status = 402;
                XA = XA_init;
                XB = XB_init;
            else
                status = 402.5;
                XA = XA_prev;
                XB = XB_prev;
            end
        end

    else
        
        if isempty(XA_prev)
            status = 403;
            XA = XA_init;
            XB = XB_init;
        else
            status = 407;
            XA = XA_prev;
            XB = XB_prev;
        end

    end
end

end
